simulink model "positionController"  (R2025b)
settings: Solver=FixedStepDiscrete  StartTime=0.0  StopTime=10.0  RelTol=1e-3
undefined symbols (not defined in the file or in its folder): controller_mode, controller_modes, controllerGains, DiscIntNeverNeededParam
libraries: simulink x4, simulink_extras x2, metux_library x1
settings Model: Creator=karadeli  LastModifiedBy=karadeli
settings OptimizationCC: DefaultParameterBehavior=Inlined  GainParamInheritBuiltInType=on  UseFloatMulNetSlope=on  InlineInvariantSignals=on  PassReuseOutputArgsAs=Individual arguments  ZeroExternalMemoryAtStartup=off  ZeroInternalMemoryAtStartup=off  NoFixptDivByZeroProtection=on  EfficientFloat2IntCast=on  LifeSpan=1  OptimizeBlockOrder=speed  DifferentSizesBufferReuse=on  EfficientTunableParamExpr=on
settings DebuggingCC: ParamSuppressDoubleToSinglePrecisionLossMsg=on  ParameterTunabilityLossMsg=none  SFUnexpectedBacktrackingDiag=warning  SFNoUnconditionalDefaultTransitionDiag=warning
settings HardwareCC: ProdBitPerPointer=32.0  ProdBitPerSizeT=32.0  ProdBitPerPtrDiffT=32.0  ProdLargestAtomicInteger=Long  ProdLargestAtomicFloat=Double  ProdWordSize=32.0  ProdLongLongMode=on  ProdHWDeviceType=ARM Compatible->ARM Cortex-M
settings SFSimCC: MATLABDynamicMemAlloc=off
settings RTWCC: SystemTargetFile=ert.tlc  GenCodeOnly=on  TemplateMakefile=ert_default_tmf  BuildConfiguration=Debug  TargetLang=C++  Description=Embedded Coder
settings CodeAppCC: ForceParamTrailComments=on  IgnoreCustomStorageClasses=off  OperatorAnnotations=on  SimulinkDataObjDesc=on  SFDataObjDesc=on  CustomSymbolStrGlobalVar=rt$N$M  CustomSymbolStrType=$N$M  CustomSymbolStrFcn=$N$M$F  CustomSymbolStrMacro=$N$M  InsertBlockDesc=on  EnableCustomComments=on
settings ERTTargetCC: RootIOFormat=Structure reference  ERTCustomFileTemplate=example_file_process.tlc  ERTFilePackagingFormat=CompactWithDataFile  TargetLangStandard=C++11 (ISO)  GenerateSampleERTMain=on  IncludeMdlTerminateFcn=off  CombineSignalStateStructs=on  SuppressErrorStatus=on  SupportAbsoluteTime=off  CodeInterfacePackaging=C++ class  SubcomponentCodeInterfacePackaging=C++ class  SupportComplex=off

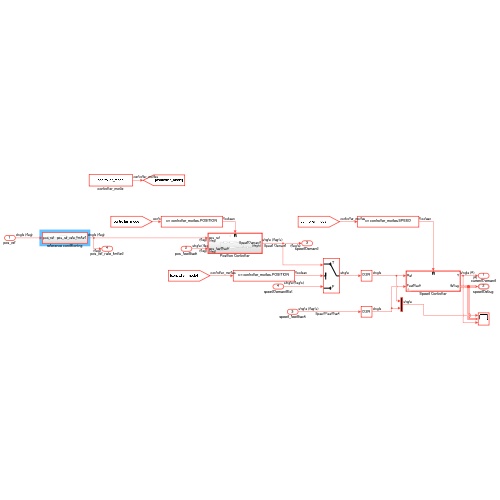
[thumbnail: Simulink's stored preview of the top-level diagram]
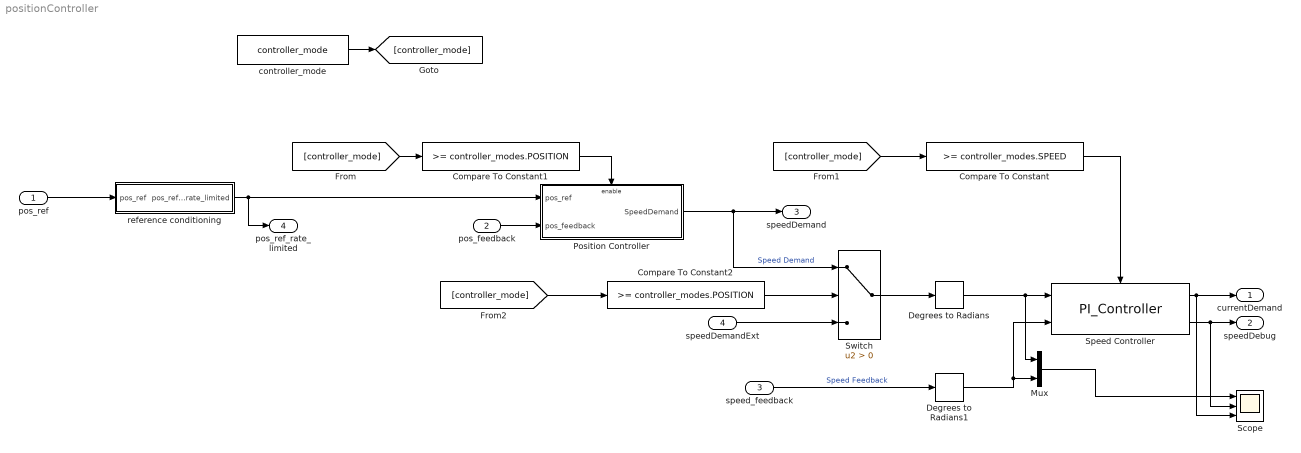
== system positionController ==
  pos_ref : Inport  OutDataTypeStr=single  Unit=deg  SampleTime=controllerGains.position.Ts  Interpolate=off
  pos_feedback : Inport  Port=2  Unit=deg  SampleTime=controllerGains.position.Ts  Interpolate=off
  speed_feedback : Inport  Port=3  Unit=deg/s  SampleTime=controllerGains.speed.Ts  Interpolate=off
  speedDemandExt : Inport  Port=4  Unit=deg/s
  Compare To Constant : simulink/Logic and Bit Operations/Compare To Constant  relop=>=  const=controller_modes.SPEED  OutDataTypeStr=boolean
  Compare To Constant1 : simulink/Logic and Bit Operations/Compare To Constant  relop=>=  const=controller_modes.POSITION  OutDataTypeStr=boolean
  Compare To Constant2 : simulink/Logic and Bit Operations/Compare To Constant  relop=>=  const=controller_modes.POSITION  OutDataTypeStr=boolean
  Degrees to Radians : simulink_extras/Transformations/Degrees to Radians
  Degrees to Radians1 : simulink_extras/Transformations/Degrees to Radians
  Mux : Mux  Inputs=2
  Position Controller : Subsystem
  Scope : Scope  NumInputPorts=3
      settings: ActiveDisplayYMinimum=-3482.2818450927725  ActiveDisplayYMaximum=28164.697982788086
  Speed Controller : metux_library/PI_Controller  Kp=controllerGains.speed.Kp  Ki=controllerGains.speed.Ki  SatMax=controllerGains.speed.SatMax  SatMin=controllerGains.speed.SatMin  Ts=controllerGains.speed.Ts  RateLimiterMax=controllerGains.speed.RateLimiterMax  RateLimiterMin=controllerGains.speed.RateLimiterMin
  Switch : Switch  Criteria=u2 > Threshold  SaturateOnIntegerOverflow=off
  controller_mode : Constant  Value=controller_mode  SampleTime=-1
  reference conditioning : Subsystem
  currentDemand : Outport  Unit=A
  speedDebug : Outport  Port=2  OutDataTypeStr=Bus: PI_debug  Unit=A  BusOutputAsStruct=on
  speedDemand : Outport  Port=3  Unit=deg/s
  pos_ref_rate_limited : Outport  Port=4  Unit=deg
  wires:
  Compare To Constant1/1 -> Position Controller/Enable
  pos_feedback/1 -> Position Controller/2(pos_feedback)
  speed_feedback/1 -> Degrees to Radians1/1  "Speed Feedback"
  Speed Controller/1 -> currentDemand/1, Scope/3
  Speed Controller/2 -> Scope/2, speedDebug/1
  Mux/1 -> Scope/1
  Compare To Constant/1 -> Speed Controller/Enable
  Position Controller/1(SpeedDemand) -> Switch/1, speedDemand/1  "Speed Demand"
  controller_mode/1 -> [controller_mode]
  [controller_mode] -> Compare To Constant1/1
  [controller_mode] -> Compare To Constant/1
  reference conditioning/1(pos_ref_rate_limited) -> pos_ref_rate_limited/1, Position Controller/1(pos_ref)
  pos_ref/1 -> reference conditioning/1(pos_ref)
  [controller_mode] -> Compare To Constant2/1
  Compare To Constant2/1 -> Switch/2
  speedDemandExt/1 -> Switch/3
  Switch/1 -> Degrees to Radians/1
  Degrees to Radians/1 -> Mux/1, Speed Controller/1
  Degrees to Radians1/1 -> Speed Controller/2, Mux/2

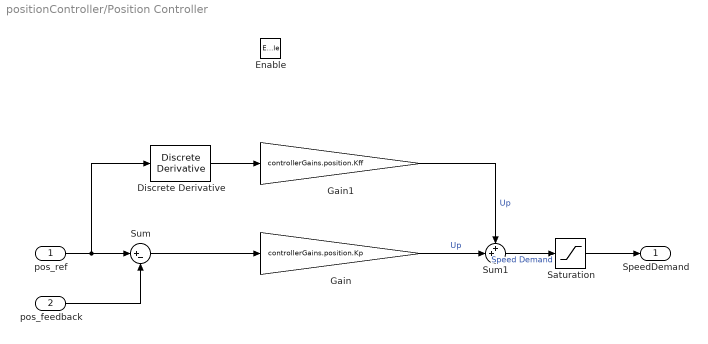
== system positionController/Position Controller ==
  pos_ref : Inport  Unit=deg
  pos_feedback : Inport  Port=2  Unit=deg
  Enable : EnablePort  StatesWhenEnabling=reset
  Discrete Derivative : simulink/Discrete/Discrete Derivative  gainval=1.0  ICPrevScaledInput=0.0  OutMin=[]  OutMax=[]  OutDataType=fixdt(1, 16)  OutScaling=2^-10  DoSatur=off
  Gain : Gain  Gain=controllerGains.position.Kp
  Gain1 : Gain  Gain=controllerGains.position.Kff
  Saturation : Saturate  UpperLimit=controllerGains.position.SatMax  LowerLimit=controllerGains.position.SatMin
  Sum : Sum  Inputs=|+-
  Sum1 : Sum  Inputs=++|
  SpeedDemand : Outport  Unit=deg/s  OutputWhenDisabled=reset  InitialOutput=[0.0]
  wires:
  Saturation/1 -> SpeedDemand/1
  pos_feedback/1 -> Sum/2
  Gain/1 -> Sum1/2  "Up"
  Sum/1 -> Gain/1
  pos_ref/1 -> Discrete Derivative/1, Sum/1
  Sum1/1 -> Saturation/1  "Speed Demand"
  Discrete Derivative/1 -> Gain1/1
  Gain1/1 -> Sum1/1  "Up"

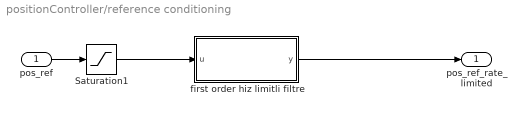
== system positionController/reference conditioning ==
  pos_ref : Inport
  Saturation1 : Saturate  UpperLimit=360*4  LowerLimit=0
  first order hiz limitli filtre : Subsystem
  pos_ref_rate_limited : Outport
  wires:
  pos_ref/1 -> Saturation1/1
  Saturation1/1 -> first order hiz limitli filtre/1(u)
  first order hiz limitli filtre/1(y) -> pos_ref_rate_limited/1

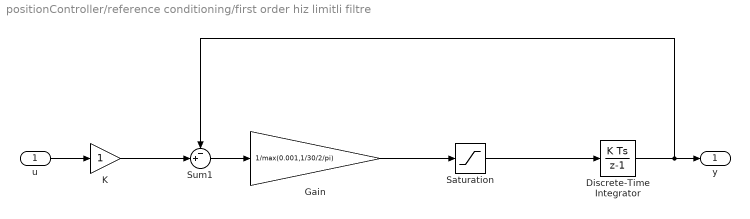
== system positionController/reference conditioning/first order hiz limitli filtre ==
  u : Inport
  Discrete-Time Integrator : DiscreteIntegrator  SampleTime=-1  ICPrevOutput=DiscIntNeverNeededParam  ICPrevScaledInput=DiscIntNeverNeededParam
  Gain : Gain  Gain=1/max(0.001,1/30/2/pi)
  K : Gain
  Saturation : Saturate  UpperLimit=2400  LowerLimit=-2400
  Sum1 : Sum  Inputs=-+|
  y : Outport  VectorParamsAs1DForOutWhenUnconnected=off
  wires:
  K/1 -> Sum1/2
  Sum1/1 -> Gain/1
  Gain/1 -> Saturation/1
  Discrete-Time Integrator/1 -> Sum1/1, y/1
  u/1 -> K/1
  Saturation/1 -> Discrete-Time Integrator/1
